simulink subsystem "sens_modelling"  (R2024a)
settings: Solver=VariableStepAuto  StartTime=0.0  StopTime=10.0  RelTol=1e-3
undefined symbols (not defined in the file or in its folder): fractalcoef, imu_sample_time
libraries: aerolibutil x3, matrix_library x1, mspsensorlib x1
settings Model: Creator=joshu  LastModifiedBy=joshu

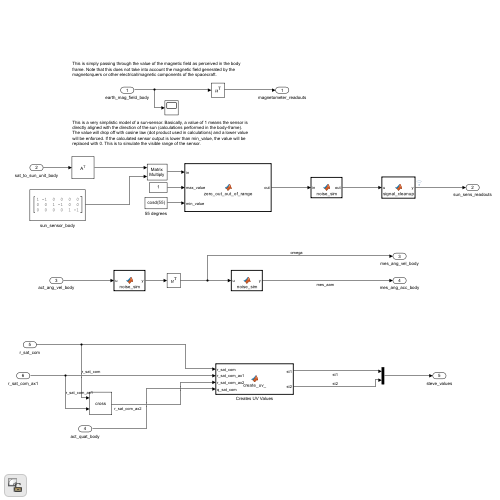
[thumbnail: Simulink's stored preview of the top-level diagram]
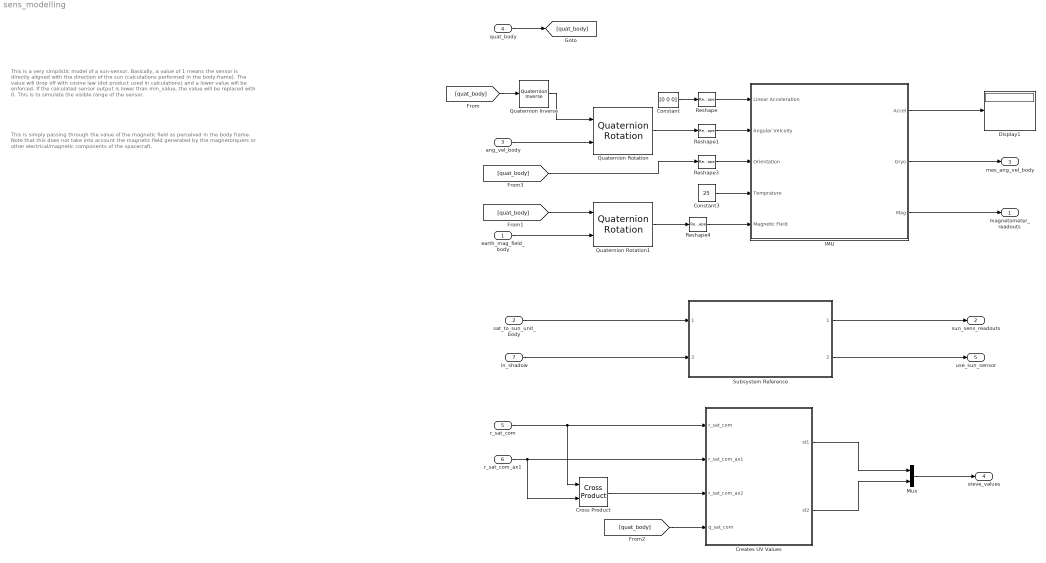
== system sens_modelling ==
  note: This is simply passing through the value of the magnetic field as perceived in the body frame. Note that this does not take into account the magnetic field generated by the magnetorquers or other electrical/magnetic components of the spacecraft.
  note: This is a very simplistic model of a sun-sensor. Basically, a value of 1 means the sensor is directly aligned with the direction of the sun (calculations performed in the body-frame). The value will drop off with cosine law (dot product used in calculations) and a lower value will be enforced. If the calculated sensor output is lower than min_value, the value will be replaced with 0. This is to simulate the visible range of the sensor.
  earth_mag_field_body : Inport
  sat_to_sun_unit_body : Inport  Port=2
  ang_vel_body : Inport  Port=3
  quat_body : Inport  Port=4
  r_sat_com : Inport  Port=5
  r_sat_com_ax1 : Inport  Port=6
  in_shadow : Inport  Port=7
  Constant : Constant  Value=[0 0 0]
  Constant3 : Constant  Value=25
  Creates UV Values : MATLAB Function  TreatAsAtomicUnit=on
  Cross Product : matrix_library/Cross Product
  Display1 : Display
  IMU : Subsystem  TreatAsAtomicUnit=on  SystemSampleTime=imu_sample_time
  Mux : Mux  Inputs=2
  Quaternion Inverse : aerolibutil/Quaternion Inverse
  Quaternion Rotation : aerolibutil/Quaternion Rotation
  Quaternion Rotation1 : aerolibutil/Quaternion Rotation
  Reshape{,1,3..4} (4 alike) : Reshape  OutputDimensionality=Row vector (2-D)
  Subsystem Reference : Subsystem  ReferencedSubsystem=sun_sensor_model
  magnetometer_readouts : Outport
  sun_sens_readouts : Outport  Port=2
  mes_ang_vel_body : Outport  Port=3
  steve_values : Outport  Port=4
  use_sun_sensor : Outport  Port=5
  wires:
  Mux/1 -> steve_values/1
  r_sat_com_ax1/1 -> Cross Product/2, Creates UV Values/2(r_sat_com_ax1)
  Cross Product/1 -> Creates UV Values/3(r_sat_com_ax2)
  r_sat_com/1 -> Creates UV Values/1(r_sat_com), Cross Product/1
  Creates UV Values/2(st2) -> Mux/2
  Creates UV Values/1(st1) -> Mux/1
  sat_to_sun_unit_body/1 -> Subsystem Reference/1
  in_shadow/1 -> Subsystem Reference/2
  Subsystem Reference/1 -> sun_sens_readouts/1
  Subsystem Reference/2 -> use_sun_sensor/1
  Constant/1 -> Reshape/1
  Constant3/1 -> IMU/4(Temprature)
  IMU/1(Accel) -> Display1/1
  IMU/3(Mag) -> magnetometer_readouts/1
  Reshape4/1 -> IMU/5(Magnetic Field)
  Reshape1/1 -> IMU/2(Angular Velcoity)
  Reshape/1 -> IMU/1(Linear Acceleration)
  earth_mag_field_body/1 -> Quaternion Rotation1/2
  Quaternion Rotation/1 -> Reshape1/1
  Quaternion Rotation1/1 -> Reshape4/1
  Reshape3/1 -> IMU/3(Orientation)
  quat_body/1 -> [quat_body]
  Quaternion Inverse/1 -> Quaternion Rotation/1
  [quat_body] -> Quaternion Inverse/1
  [quat_body] -> Quaternion Rotation1/1
  [quat_body] -> Creates UV Values/4(q_sat_com)
  [quat_body] -> Reshape3/1
  IMU/2(Gryo) -> mes_ang_vel_body/1
  ang_vel_body/1 -> Quaternion Rotation/2

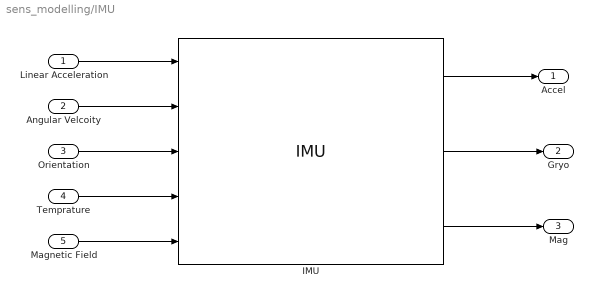
== system sens_modelling/IMU ==
  Linear Acceleration : Inport
  Angular Velcoity : Inport  Port=2
  Orientation : Inport  Port=3
  Temprature : Inport  Port=4
  Magnetic Field : Inport  Port=5
  IMU : mspsensorlib/IMU  DispRefFrame=NED  TemperaturePort=on  Temperature=25  MagneticFieldPort=on  MagneticFieldNED=[ 27.5550, -2.4169, -16.0849 ]  MagneticFieldENU=[ -2.4169, 27.5550, 16.0849 ]  SeedDouble=67  SimulateUsing=Interpreted execution  AccelParamsMeasurementRange=Inf  AccelParamsResolution=0  AccelParamsConstantBias=[ 0, 0, 0 ]  AccelParamsAxesMisalignment=[ 100, 0, 0; 0, 100, 0; 0, 0, 100 ]  AccelParamsNoiseDensity=[ 0, 0, 0 ]  AccelParamsBiasInstability=[ 0, 0, 0 ]  AccelParamsBiasInstabilityNumerator=fractalcoef().Numerator  AccelParamsBiasInstabilityDenominator=fractalcoef().Denominator  AccelParamsRandomWalk=[ 0, 0, 0 ]  AccelParamsNoiseType=double-sided  AccelParamsTemperatureBias=[ 0, 0, 0 ]  AccelParamsTemperatureScaleFactor=[ 0, 0, 0 ]  GyroParamsMeasurementRange=Inf  GyroParamsResolution=0  GyroParamsConstantBias=[ 0, 0, 0 ]  GyroParamsAxesMisalignment=[ 100, 0, 0; 0, 100, 0; 0, 0, 100 ]  GyroParamsAccelerationBias=[ 0, 0, 0 ]  GyroParamsNoiseDensity=[ 0, 0, 0 ]  GyroParamsBiasInstability=[ 0, 0, 0 ]  GyroParamsBiasInstabilityNumerator=fractalcoef().Numerator  GyroParamsBiasInstabilityDenominator=fractalcoef().Denominator  GyroParamsRandomWalk=[ 0, 0, 0 ]  GyroParamsNoiseType=double-sided  GyroParamsTemperatureBias=[ 0, 0, 0 ]  GyroParamsTemperatureScaleFactor=[ 0, 0, 0 ]  MagParamsMeasurementRange=Inf  MagParamsResolution=0  MagParamsConstantBias=[ 0, 0, 0 ]  MagParamsAxesMisalignment=[ 100, 0, 0; 0, 100, 0; 0, 0, 100 ]  MagParamsNoiseDensity=[ 0, 0, 0 ]  MagParamsBiasInstability=[ 0, 0, 0 ]  MagParamsBiasInstabilityNumerator=fractalcoef().Numerator  MagParamsBiasInstabilityDenominator=fractalcoef().Denominator  MagParamsRandomWalk=[ 0, 0, 0 ]  MagParamsNoiseType=double-sided  MagParamsTemperatureBias=[ 0, 0, 0 ]  MagParamsTemperatureScaleFactor=[ 0, 0, 0 ]
  Accel : Outport
  Gryo : Outport  Port=2
  Mag : Outport  Port=3
  wires:
  IMU/3 -> Mag/1
  IMU/2 -> Gryo/1
  Magnetic Field/1 -> IMU/5
  Temprature/1 -> IMU/4
  Orientation/1 -> IMU/3
  Angular Velcoity/1 -> IMU/2
  IMU/1 -> Accel/1
  Linear Acceleration/1 -> IMU/1

== matlab function sens_modelling/Creates UV Values ==
  data: r_sat_com input; st1 output; r_sat_com_ax1 input; r_sat_com_ax2 input; q_sat_com input; st2 output
function [st1,st2] = create_uv_(r_sat_com,r_sat_com_ax1, ...
                                r_sat_com_ax2,q_sat_com)

    [st1,st2] = create_uv(r_sat_com,r_sat_com_ax1, ...
                           r_sat_com_ax2,q_sat_com);

end
